simulink model "application"  (R2021b)
settings: Solver=FixedStepAuto  StartTime=0.0  StopTime=10.0  FixedStep=sampleTime  RelTol=1e-3
undefined symbols (not defined in the file or in its folder): AEMACE10_STBY, AEMACE8_STBY
libraries: simulink x10, EMACE_APP x6, AIL_STATE_MACHINE_LIB x2, AEMACE10_IN x1, AEMACE10_INSTRUMENTATION x1, AEMACE10_OUT x1, AEMACE8_IN x1, AEMACE8_INSTRUMENTATION x1, AEMACE8_OUT x1, SEMACE1_IN x1, SEMACE1_INSTRUMENTATION x1, SEMACE1_OUT x1
(part 2 of 2)

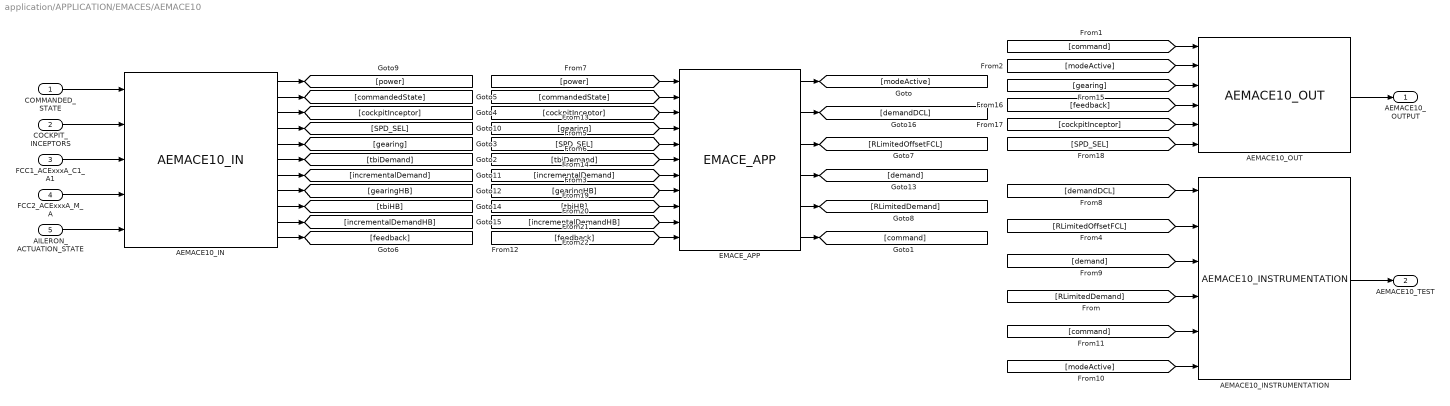
== system application/APPLICATION/EMACES/AEMACE10 ==
  COMMANDED_STATE : Inport
  COCKPIT_INCEPTORS : Inport  Port=2
  FCC1_ACExxxA_C1_A1 : Inport  Port=3
  FCC2_ACExxxA_M_A : Inport  Port=4
  AILERON_ACTUATION_STATE : Inport  Port=5
  AEMACE10_IN : AEMACE10_IN/AEMACE10_IN  SystemSampleTime=-1  VariantActivationTime=update diagram  Latency=0  AutoFrameSizeCalculation=off
  AEMACE10_INSTRUMENTATION : AEMACE10_INSTRUMENTATION/AEMACE10_INSTRUMENTATION  SystemSampleTime=-1  VariantActivationTime=update diagram  Latency=0  AutoFrameSizeCalculation=off
  AEMACE10_OUT : AEMACE10_OUT/AEMACE10_OUT  SystemSampleTime=-1  VariantActivationTime=update diagram  Latency=0  AutoFrameSizeCalculation=off
  EMACE_APP : EMACE_APP/EMACE_APP  SystemSampleTime=-1  VariantActivationTime=update diagram  Latency=0  AutoFrameSizeCalculation=off
      link override From10: GotoTag=command
  AEMACE10_OUTPUT : Outport
  AEMACE10_TEST : Outport  Port=2
  wires:
  COMMANDED_STATE/1 -> AEMACE10_IN/1
  COCKPIT_INCEPTORS/1 -> AEMACE10_IN/2
  FCC1_ACExxxA_C1_A1/1 -> AEMACE10_IN/3
  AILERON_ACTUATION_STATE/1 -> AEMACE10_IN/5
  [command] -> AEMACE10_OUT/1
  [modeActive] -> AEMACE10_OUT/2
  AEMACE10_OUT/1 -> AEMACE10_OUTPUT/1
  [demandDCL] -> AEMACE10_INSTRUMENTATION/1
  AEMACE10_INSTRUMENTATION/1 -> AEMACE10_TEST/1
  EMACE_APP/1 -> [modeActive]
  EMACE_APP/2 -> [demandDCL]
  EMACE_APP/6 -> [command]
  EMACE_APP/4 -> [demand]
  EMACE_APP/3 -> [RLimitedOffsetFCL]
  EMACE_APP/5 -> [RLimitedDemand]
  [modeActive] -> AEMACE10_INSTRUMENTATION/6
  [command] -> AEMACE10_INSTRUMENTATION/5
  [RLimitedDemand] -> AEMACE10_INSTRUMENTATION/4
  [demand] -> AEMACE10_INSTRUMENTATION/3
  [RLimitedOffsetFCL] -> AEMACE10_INSTRUMENTATION/2
  AEMACE10_IN/1 -> [power]
  AEMACE10_IN/4 -> [SPD_SEL]
  AEMACE10_IN/5 -> [gearing]
  AEMACE10_IN/6 -> [tbiDemand]
  AEMACE10_IN/11 -> [feedback]
  AEMACE10_IN/2 -> [commandedState]
  AEMACE10_IN/3 -> [cockpitInceptor]
  [power] -> EMACE_APP/1
  [commandedState] -> EMACE_APP/2
  [cockpitInceptor] -> EMACE_APP/3
  [gearing] -> EMACE_APP/4
  [SPD_SEL] -> EMACE_APP/5
  [tbiDemand] -> EMACE_APP/6
  [feedback] -> EMACE_APP/11
  [gearing] -> AEMACE10_OUT/3
  [feedback] -> AEMACE10_OUT/4
  [cockpitInceptor] -> AEMACE10_OUT/5
  [SPD_SEL] -> AEMACE10_OUT/6
  FCC2_ACExxxA_M_A/1 -> AEMACE10_IN/4
  AEMACE10_IN/7 -> [incrementalDemand]
  AEMACE10_IN/8 -> [gearingHB]
  AEMACE10_IN/9 -> [tbiHB]
  AEMACE10_IN/10 -> [incrementalDemandHB]
  [incrementalDemand] -> EMACE_APP/7
  [gearingHB] -> EMACE_APP/8
  [incrementalDemandHB] -> EMACE_APP/10
  [tbiHB] -> EMACE_APP/9

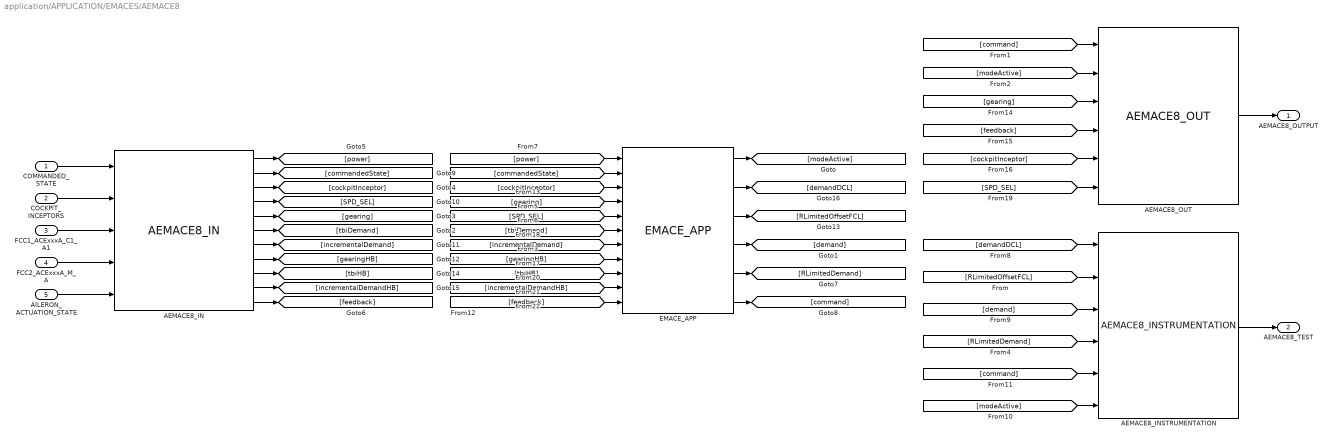
== system application/APPLICATION/EMACES/AEMACE8 ==
  COMMANDED_STATE : Inport
  COCKPIT_INCEPTORS : Inport  Port=2
  FCC1_ACExxxA_C1_A1 : Inport  Port=3
  FCC2_ACExxxA_M_A : Inport  Port=4
  AILERON_ACTUATION_STATE : Inport  Port=5
  AEMACE8_IN : AEMACE8_IN/AEMACE8_IN  SystemSampleTime=-1  VariantActivationTime=update diagram  Latency=0  AutoFrameSizeCalculation=off
      link override Rate Limiter: RisingSlewLimit=dataAEMACE.rateLimiterGearing  FallingSlewLimit=-dataAEMACE.rateLimiterGearing
  AEMACE8_INSTRUMENTATION : AEMACE8_INSTRUMENTATION/AEMACE8_INSTRUMENTATION  SystemSampleTime=-1  VariantActivationTime=update diagram  Latency=0  AutoFrameSizeCalculation=off
  AEMACE8_OUT : AEMACE8_OUT/AEMACE8_OUT  SystemSampleTime=-1  VariantActivationTime=update diagram  Latency=0  AutoFrameSizeCalculation=off
  EMACE_APP : EMACE_APP/EMACE_APP  SystemSampleTime=-1  VariantActivationTime=update diagram  Latency=0  AutoFrameSizeCalculation=off
  AEMACE8_OUTPUT : Outport
  AEMACE8_TEST : Outport  Port=2
  wires:
  COMMANDED_STATE/1 -> AEMACE8_IN/1
  COCKPIT_INCEPTORS/1 -> AEMACE8_IN/2
  FCC1_ACExxxA_C1_A1/1 -> AEMACE8_IN/3
  AILERON_ACTUATION_STATE/1 -> AEMACE8_IN/5
  AEMACE8_OUT/1 -> AEMACE8_OUTPUT/1
  [demandDCL] -> AEMACE8_INSTRUMENTATION/1
  AEMACE8_INSTRUMENTATION/1 -> AEMACE8_TEST/1
  EMACE_APP/1 -> [modeActive]
  EMACE_APP/2 -> [demandDCL]
  EMACE_APP/3 -> [RLimitedOffsetFCL]
  EMACE_APP/4 -> [demand]
  EMACE_APP/5 -> [RLimitedDemand]
  EMACE_APP/6 -> [command]
  [RLimitedOffsetFCL] -> AEMACE8_INSTRUMENTATION/2
  [demand] -> AEMACE8_INSTRUMENTATION/3
  [RLimitedDemand] -> AEMACE8_INSTRUMENTATION/4
  [command] -> AEMACE8_INSTRUMENTATION/5
  [modeActive] -> AEMACE8_INSTRUMENTATION/6
  [power] -> EMACE_APP/1
  [commandedState] -> EMACE_APP/2
  [cockpitInceptor] -> EMACE_APP/3
  [gearing] -> EMACE_APP/4
  [command] -> AEMACE8_OUT/1
  [modeActive] -> AEMACE8_OUT/2
  [gearing] -> AEMACE8_OUT/3
  [feedback] -> AEMACE8_OUT/4
  [cockpitInceptor] -> AEMACE8_OUT/5
  [SPD_SEL] -> EMACE_APP/5
  [tbiDemand] -> EMACE_APP/6
  [feedback] -> EMACE_APP/11
  [SPD_SEL] -> AEMACE8_OUT/6
  FCC2_ACExxxA_M_A/1 -> AEMACE8_IN/4
  AEMACE8_IN/1 -> [power]
  AEMACE8_IN/2 -> [commandedState]
  AEMACE8_IN/3 -> [cockpitInceptor]
  AEMACE8_IN/4 -> [SPD_SEL]
  AEMACE8_IN/5 -> [gearing]
  AEMACE8_IN/6 -> [tbiDemand]
  AEMACE8_IN/11 -> [feedback]
  AEMACE8_IN/7 -> [incrementalDemand]
  AEMACE8_IN/8 -> [gearingHB]
  AEMACE8_IN/9 -> [tbiHB]
  AEMACE8_IN/10 -> [incrementalDemandHB]
  [incrementalDemand] -> EMACE_APP/7
  [gearingHB] -> EMACE_APP/8
  [tbiHB] -> EMACE_APP/9
  [incrementalDemandHB] -> EMACE_APP/10

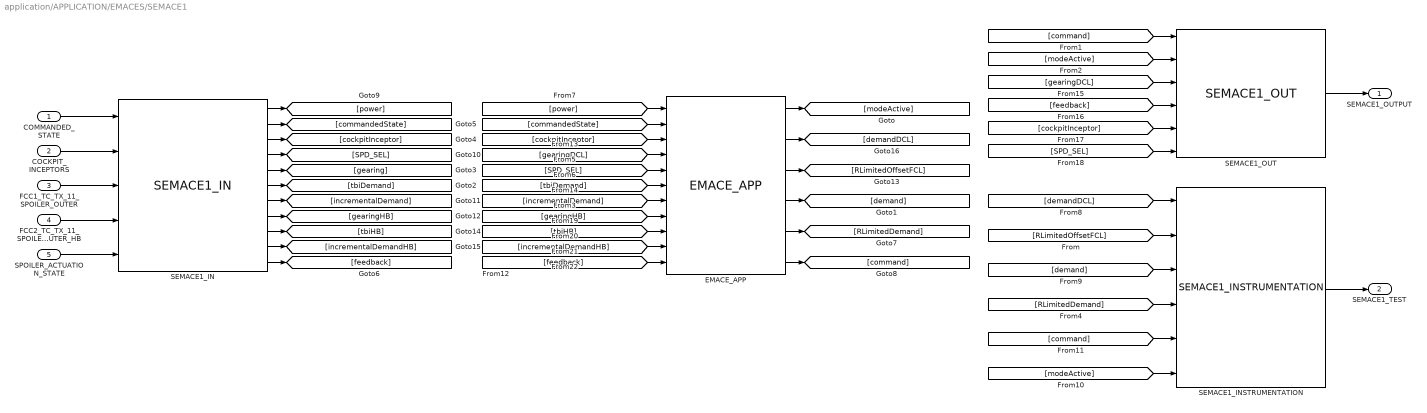
== system application/APPLICATION/EMACES/SEMACE1 ==
  COMMANDED_STATE : Inport
  COCKPIT_INCEPTORS : Inport  Port=2
  FCC1_TC_TX_11_SPOILER_OUTER : Inport  Port=3  OutDataTypeStr=Bus: FCC1_TC_TX_11_SPOILER_OUTER
  FCC2_TC_TX_11_SPOILER_OUTER_HB : Inport  Port=4  OutDataTypeStr=Bus: FCC2_TC_TX_11_SPOILER_OUTER_HB
  SPOILER_ACTUATION_STATE : Inport  Port=5  OutDataTypeStr=Bus: SPOILER_ACTUATION_STATE
  EMACE_APP : EMACE_APP/EMACE_APP  SystemSampleTime=-1  VariantActivationTime=update diagram  Latency=0  AutoFrameSizeCalculation=off
  SEMACE1_IN : SEMACE1_IN/SEMACE1_IN  SystemSampleTime=-1  VariantActivationTime=update diagram  Latency=0  AutoFrameSizeCalculation=off
  SEMACE1_INSTRUMENTATION : SEMACE1_INSTRUMENTATION/SEMACE1_INSTRUMENTATION  SystemSampleTime=-1  VariantActivationTime=update diagram  Latency=0  AutoFrameSizeCalculation=off
  SEMACE1_OUT : SEMACE1_OUT/SEMACE1_OUT  SystemSampleTime=-1  VariantActivationTime=update diagram  Latency=0  AutoFrameSizeCalculation=off
  SEMACE1_OUTPUT : Outport
  SEMACE1_TEST : Outport  Port=2
  wires:
  COMMANDED_STATE/1 -> SEMACE1_IN/1
  COCKPIT_INCEPTORS/1 -> SEMACE1_IN/2
  FCC1_TC_TX_11_SPOILER_OUTER/1 -> SEMACE1_IN/3
  SPOILER_ACTUATION_STATE/1 -> SEMACE1_IN/5
  [command] -> SEMACE1_OUT/1
  [modeActive] -> SEMACE1_OUT/2
  SEMACE1_OUT/1 -> SEMACE1_OUTPUT/1
  [demandDCL] -> SEMACE1_INSTRUMENTATION/1
  SEMACE1_INSTRUMENTATION/1 -> SEMACE1_TEST/1
  EMACE_APP/1 -> [modeActive]
  EMACE_APP/2 -> [demandDCL]
  EMACE_APP/3 -> [RLimitedOffsetFCL]
  EMACE_APP/4 -> [demand]
  EMACE_APP/5 -> [RLimitedDemand]
  EMACE_APP/6 -> [command]
  [RLimitedOffsetFCL] -> SEMACE1_INSTRUMENTATION/2
  [demand] -> SEMACE1_INSTRUMENTATION/3
  [RLimitedDemand] -> SEMACE1_INSTRUMENTATION/4
  [command] -> SEMACE1_INSTRUMENTATION/5
  [modeActive] -> SEMACE1_INSTRUMENTATION/6
  SEMACE1_IN/4 -> [SPD_SEL]
  SEMACE1_IN/5 -> [gearing]
  SEMACE1_IN/6 -> [tbiDemand]
  SEMACE1_IN/11 -> [feedback]
  SEMACE1_IN/1 -> [power]
  SEMACE1_IN/2 -> [commandedState]
  SEMACE1_IN/3 -> [cockpitInceptor]
  [power] -> EMACE_APP/1
  [commandedState] -> EMACE_APP/2
  [cockpitInceptor] -> EMACE_APP/3
  [gearingDCL] -> EMACE_APP/4
  [SPD_SEL] -> EMACE_APP/5
  [tbiDemand] -> EMACE_APP/6
  [feedback] -> EMACE_APP/11
  [gearingDCL] -> SEMACE1_OUT/3
  [feedback] -> SEMACE1_OUT/4
  [cockpitInceptor] -> SEMACE1_OUT/5
  [SPD_SEL] -> SEMACE1_OUT/6
  FCC2_TC_TX_11_SPOILER_OUTER_HB/1 -> SEMACE1_IN/4
  SEMACE1_IN/7 -> [incrementalDemand]
  SEMACE1_IN/8 -> [gearingHB]
  SEMACE1_IN/9 -> [tbiHB]
  SEMACE1_IN/10 -> [incrementalDemandHB]
  [incrementalDemandHB] -> EMACE_APP/10
  [tbiHB] -> EMACE_APP/9
  [gearingHB] -> EMACE_APP/8
  [incrementalDemand] -> EMACE_APP/7

== system application/APPLICATION/EMACES/SEMACE2 ==
  COMMANDED_STATE : Inport
  COCKPIT_INCEPTORS : Inport  Port=2
  FCC1_TC_TX_12_SPOILER_INNER : Inport  Port=3  OutDataTypeStr=Bus: FCC1_TC_TX_12_SPOILER_INNER
  FCC2_TC_TX_12_SPOILER_INNER_HB : Inport  Port=4  OutDataTypeStr=Bus: FCC2_TC_TX_12_SPOILER_INNER_HB
  SPOILER_ACTUATION_STATE : Inport  Port=5  OutDataTypeStr=Bus: SPOILER_ACTUATION_STATE
  EMACE_APP : EMACE_APP/EMACE_APP  SystemSampleTime=-1  VariantActivationTime=update diagram  Latency=0  AutoFrameSizeCalculation=off
  SEMACE2_IN : SEMACE2_IN/SEMACE2_IN  SystemSampleTime=-1  VariantActivationTime=update diagram  Latency=0  AutoFrameSizeCalculation=off
  SEMACE2_INSTRUMENTATION : SEMACE2_INSTRUMENTATION/SEMACE2_INSTRUMENTATION  SystemSampleTime=-1  VariantActivationTime=update diagram  Latency=0  AutoFrameSizeCalculation=off
  SEMACE2_OUT : SEMACE2_OUT/SEMACE2_OUT  SystemSampleTime=-1  VariantActivationTime=update diagram  Latency=0  AutoFrameSizeCalculation=off
  SEMACE2_OUTPUT : Outport
  SEMACE2_TEST : Outport  Port=2
  wires:
  [modeActive] -> SEMACE2_INSTRUMENTATION/6
  [command] -> SEMACE2_INSTRUMENTATION/5
  [RLimitedDemand] -> SEMACE2_INSTRUMENTATION/4
  [demand] -> SEMACE2_INSTRUMENTATION/3
  [RLimitedOffsetFCL] -> SEMACE2_INSTRUMENTATION/2
  EMACE_APP/6 -> [command]
  EMACE_APP/5 -> [RLimitedDemand]
  EMACE_APP/4 -> [demand]
  EMACE_APP/3 -> [RLimitedOffsetFCL]
  EMACE_APP/2 -> [demandDCL]
  EMACE_APP/1 -> [modeActive]
  SEMACE2_INSTRUMENTATION/1 -> SEMACE2_TEST/1
  [demandDCL] -> SEMACE2_INSTRUMENTATION/1
  SEMACE2_OUT/1 -> SEMACE2_OUTPUT/1
  [modeActive] -> SEMACE2_OUT/2
  [command] -> SEMACE2_OUT/1
  SPOILER_ACTUATION_STATE/1 -> SEMACE2_IN/5
  FCC1_TC_TX_12_SPOILER_INNER/1 -> SEMACE2_IN/3
  COCKPIT_INCEPTORS/1 -> SEMACE2_IN/2
  COMMANDED_STATE/1 -> SEMACE2_IN/1
  SEMACE2_IN/7 -> [feedback]
  SEMACE2_IN/1 -> [power]
  SEMACE2_IN/2 -> [commandedState]
  SEMACE2_IN/3 -> [cockpitInceptor]
  SEMACE2_IN/4 -> [SPD_SEL]
  SEMACE2_IN/5 -> [gearingDCL]
  SEMACE2_IN/6 -> [offsetFCL]
  [power] -> EMACE_APP/1
  [commandedState] -> EMACE_APP/2
  [cockpitInceptor] -> EMACE_APP/3
  [gearingDCL] -> EMACE_APP/4
  [SPD_SEL] -> EMACE_APP/5
  [offsetFCL] -> EMACE_APP/6
  [feedback] -> EMACE_APP/7
  [gearingDCL] -> SEMACE2_OUT/3
  [feedback] -> SEMACE2_OUT/4
  [cockpitInceptor] -> SEMACE2_OUT/5
  [SPD_SEL] -> SEMACE2_OUT/6
  FCC2_TC_TX_12_SPOILER_INNER_HB/1 -> SEMACE2_IN/4

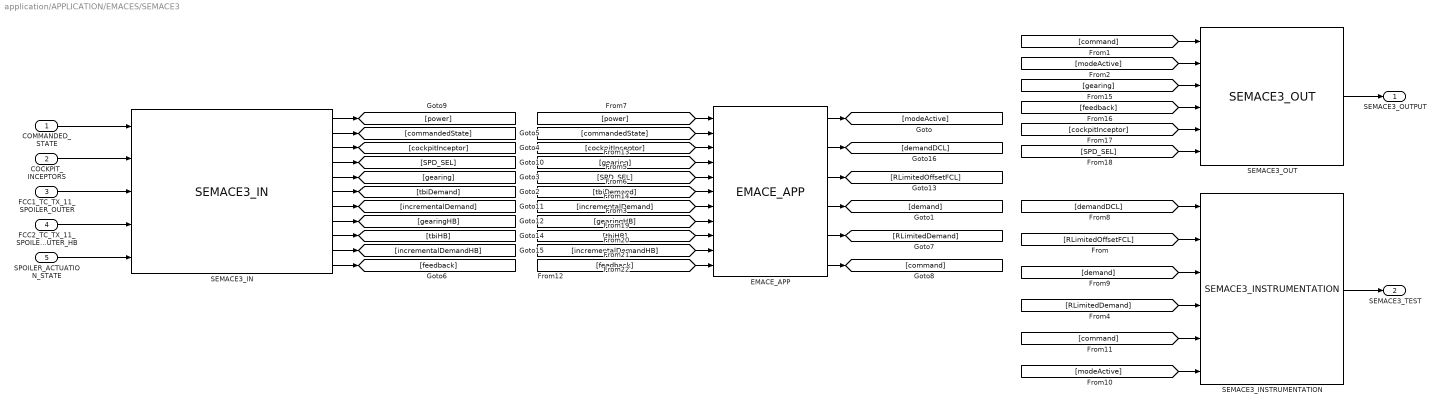
== system application/APPLICATION/EMACES/SEMACE3 ==
  COMMANDED_STATE : Inport
  COCKPIT_INCEPTORS : Inport  Port=2
  FCC1_TC_TX_11_SPOILER_OUTER : Inport  Port=3  OutDataTypeStr=Bus: FCC1_TC_TX_11_SPOILER_OUTER
  FCC2_TC_TX_11_SPOILER_OUTER_HB : Inport  Port=4  OutDataTypeStr=Bus: FCC2_TC_TX_11_SPOILER_OUTER_HB
  SPOILER_ACTUATION_STATE : Inport  Port=5  OutDataTypeStr=Bus: SPOILER_ACTUATION_STATE
  EMACE_APP : EMACE_APP/EMACE_APP  SystemSampleTime=-1  VariantActivationTime=update diagram  Latency=0  AutoFrameSizeCalculation=off
  SEMACE3_IN : SEMACE3_IN/SEMACE3_IN  SystemSampleTime=-1  VariantActivationTime=update diagram  Latency=0  AutoFrameSizeCalculation=off
  SEMACE3_INSTRUMENTATION : SEMACE3_INSTRUMENTATION/SEMACE3_INSTRUMENTATION  SystemSampleTime=-1  VariantActivationTime=update diagram  Latency=0  AutoFrameSizeCalculation=off
  SEMACE3_OUT : SEMACE3_OUT/SEMACE3_OUT  SystemSampleTime=-1  VariantActivationTime=update diagram  Latency=0  AutoFrameSizeCalculation=off
  SEMACE3_OUTPUT : Outport
  SEMACE3_TEST : Outport  Port=2
  wires:
  [modeActive] -> SEMACE3_INSTRUMENTATION/6
  [command] -> SEMACE3_INSTRUMENTATION/5
  [RLimitedDemand] -> SEMACE3_INSTRUMENTATION/4
  [demand] -> SEMACE3_INSTRUMENTATION/3
  [RLimitedOffsetFCL] -> SEMACE3_INSTRUMENTATION/2
  EMACE_APP/6 -> [command]
  EMACE_APP/5 -> [RLimitedDemand]
  EMACE_APP/4 -> [demand]
  EMACE_APP/3 -> [RLimitedOffsetFCL]
  EMACE_APP/2 -> [demandDCL]
  EMACE_APP/1 -> [modeActive]
  SEMACE3_INSTRUMENTATION/1 -> SEMACE3_TEST/1
  [demandDCL] -> SEMACE3_INSTRUMENTATION/1
  SEMACE3_OUT/1 -> SEMACE3_OUTPUT/1
  [modeActive] -> SEMACE3_OUT/2
  [command] -> SEMACE3_OUT/1
  SPOILER_ACTUATION_STATE/1 -> SEMACE3_IN/5
  FCC1_TC_TX_11_SPOILER_OUTER/1 -> SEMACE3_IN/3
  COCKPIT_INCEPTORS/1 -> SEMACE3_IN/2
  COMMANDED_STATE/1 -> SEMACE3_IN/1
  SEMACE3_IN/11 -> [feedback]
  SEMACE3_IN/1 -> [power]
  SEMACE3_IN/2 -> [commandedState]
  SEMACE3_IN/3 -> [cockpitInceptor]
  SEMACE3_IN/4 -> [SPD_SEL]
  SEMACE3_IN/5 -> [gearing]
  SEMACE3_IN/6 -> [tbiDemand]
  [power] -> EMACE_APP/1
  [commandedState] -> EMACE_APP/2
  [cockpitInceptor] -> EMACE_APP/3
  [gearing] -> EMACE_APP/4
  [SPD_SEL] -> EMACE_APP/5
  [tbiDemand] -> EMACE_APP/6
  [feedback] -> EMACE_APP/11
  [gearing] -> SEMACE3_OUT/3
  [feedback] -> SEMACE3_OUT/4
  [cockpitInceptor] -> SEMACE3_OUT/5
  [SPD_SEL] -> SEMACE3_OUT/6
  FCC2_TC_TX_11_SPOILER_OUTER_HB/1 -> SEMACE3_IN/4
  SEMACE3_IN/7 -> [incrementalDemand]
  SEMACE3_IN/8 -> [gearingHB]
  SEMACE3_IN/9 -> [tbiHB]
  SEMACE3_IN/10 -> [incrementalDemandHB]
  [incrementalDemand] -> EMACE_APP/7
  [gearingHB] -> EMACE_APP/8
  [tbiHB] -> EMACE_APP/9
  [incrementalDemandHB] -> EMACE_APP/10

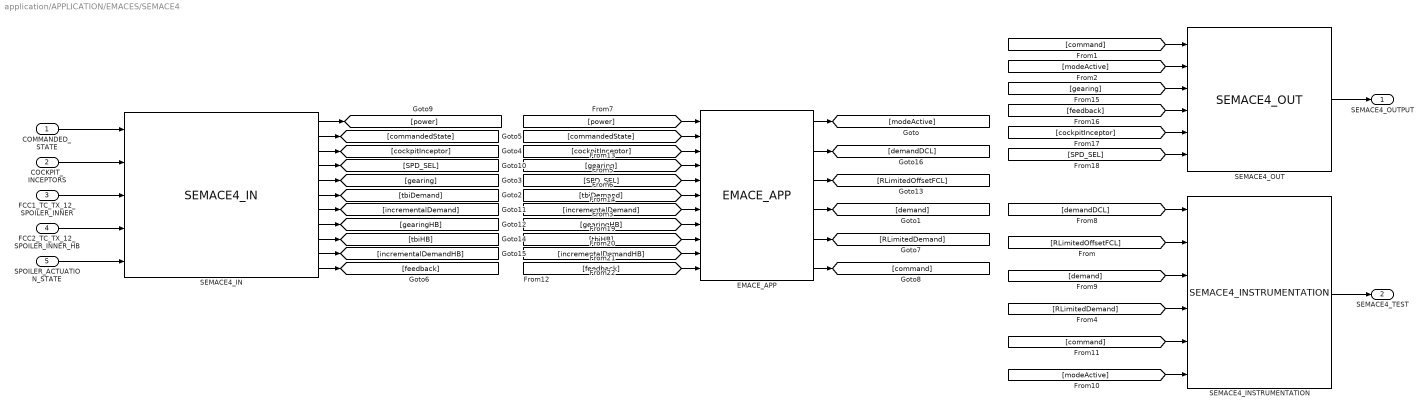
== system application/APPLICATION/EMACES/SEMACE4 ==
  COMMANDED_STATE : Inport
  COCKPIT_INCEPTORS : Inport  Port=2
  FCC1_TC_TX_12_SPOILER_INNER : Inport  Port=3  OutDataTypeStr=Bus: FCC1_TC_TX_12_SPOILER_INNER
  FCC2_TC_TX_12_SPOILER_INNER_HB : Inport  Port=4  OutDataTypeStr=Bus: FCC2_TC_TX_12_SPOILER_INNER_HB
  SPOILER_ACTUATION_STATE : Inport  Port=5  OutDataTypeStr=Bus: SPOILER_ACTUATION_STATE
  EMACE_APP : EMACE_APP/EMACE_APP  SystemSampleTime=-1  VariantActivationTime=update diagram  Latency=0  AutoFrameSizeCalculation=off
  SEMACE4_IN : SEMACE4_IN/SEMACE4_IN  SystemSampleTime=-1  VariantActivationTime=update diagram  Latency=0  AutoFrameSizeCalculation=off
  SEMACE4_INSTRUMENTATION : SEMACE4_INSTRUMENTATION/SEMACE4_INSTRUMENTATION  SystemSampleTime=-1  VariantActivationTime=update diagram  Latency=0  AutoFrameSizeCalculation=off
  SEMACE4_OUT : SEMACE4_OUT/SEMACE4_OUT  SystemSampleTime=-1  VariantActivationTime=update diagram  Latency=0  AutoFrameSizeCalculation=off
  SEMACE4_OUTPUT : Outport
  SEMACE4_TEST : Outport  Port=2
  wires:
  COMMANDED_STATE/1 -> SEMACE4_IN/1
  COCKPIT_INCEPTORS/1 -> SEMACE4_IN/2
  FCC1_TC_TX_12_SPOILER_INNER/1 -> SEMACE4_IN/3
  SPOILER_ACTUATION_STATE/1 -> SEMACE4_IN/5
  [command] -> SEMACE4_OUT/1
  [modeActive] -> SEMACE4_OUT/2
  SEMACE4_OUT/1 -> SEMACE4_OUTPUT/1
  [demandDCL] -> SEMACE4_INSTRUMENTATION/1
  SEMACE4_INSTRUMENTATION/1 -> SEMACE4_TEST/1
  EMACE_APP/1 -> [modeActive]
  EMACE_APP/2 -> [demandDCL]
  EMACE_APP/3 -> [RLimitedOffsetFCL]
  EMACE_APP/4 -> [demand]
  EMACE_APP/5 -> [RLimitedDemand]
  EMACE_APP/6 -> [command]
  [RLimitedOffsetFCL] -> SEMACE4_INSTRUMENTATION/2
  [demand] -> SEMACE4_INSTRUMENTATION/3
  [RLimitedDemand] -> SEMACE4_INSTRUMENTATION/4
  [command] -> SEMACE4_INSTRUMENTATION/5
  [modeActive] -> SEMACE4_INSTRUMENTATION/6
  SEMACE4_IN/3 -> [cockpitInceptor]
  SEMACE4_IN/4 -> [SPD_SEL]
  SEMACE4_IN/5 -> [gearing]
  SEMACE4_IN/6 -> [tbiDemand]
  SEMACE4_IN/11 -> [feedback]
  SEMACE4_IN/1 -> [power]
  SEMACE4_IN/2 -> [commandedState]
  [power] -> EMACE_APP/1
  [commandedState] -> EMACE_APP/2
  [cockpitInceptor] -> EMACE_APP/3
  [gearing] -> EMACE_APP/4
  [SPD_SEL] -> EMACE_APP/5
  [tbiDemand] -> EMACE_APP/6
  [feedback] -> EMACE_APP/11
  [gearing] -> SEMACE4_OUT/3
  [feedback] -> SEMACE4_OUT/4
  [cockpitInceptor] -> SEMACE4_OUT/5
  [SPD_SEL] -> SEMACE4_OUT/6
  FCC2_TC_TX_12_SPOILER_INNER_HB/1 -> SEMACE4_IN/4
  SEMACE4_IN/7 -> [incrementalDemand]
  SEMACE4_IN/8 -> [gearingHB]
  SEMACE4_IN/9 -> [tbiHB]
  SEMACE4_IN/10 -> [incrementalDemandHB]
  [incrementalDemand] -> EMACE_APP/7
  [gearingHB] -> EMACE_APP/8
  [tbiHB] -> EMACE_APP/9
  [incrementalDemandHB] -> EMACE_APP/10

== system application/APPLICATION/Subsystem/GENERATOR_STATE_CMD_LH_AIL ==
  LH_AIL_STATE : Inport
  Compare To Constant : simulink/Logic and Bit Operations/Compare To Constant  relop===  const=2  OutDataTypeStr=boolean
  Compare To Constant3 : simulink/Logic and Bit Operations/Compare To Constant  relop===  const=1  OutDataTypeStr=boolean
  Compare To Constant6 : simulink/Logic and Bit Operations/Compare To Constant  relop===  const=1  OutDataTypeStr=boolean
  Compare To Constant7 : simulink/Logic and Bit Operations/Compare To Constant  relop===  const=2  OutDataTypeStr=boolean
  Constant : Constant  OutDataTypeStr=boolean
  Constant1 : Constant  Value=0  OutDataTypeStr=boolean
  Constant2 : Constant  OutDataTypeStr=boolean
  Constant3 : Constant  Value=0  OutDataTypeStr=boolean
  Delay2 : Delay  DelayLength=1
  Delay3 : Delay  DelayLength=1
  Switch{,1..3} (4 alike) : Switch  Criteria=u2 > Threshold
  AEMACE8_CMD_STATE : Outport
  ACE9_CMD_STATE : Outport  Port=2
  wires:
  Constant/1 -> Switch/1
  Compare To Constant6/1 -> Switch2/2
  Switch/1 -> AEMACE8_CMD_STATE/1, Delay2/1
  Compare To Constant/1 -> Switch/2
  LH_AIL_STATE/1 -> Compare To Constant7/1, Compare To Constant6/1, Compare To Constant3/1, Compare To Constant/1
  Delay2/1 -> Switch1/3
  Switch1/1 -> Switch/3
  Constant3/1 -> Switch3/1
  Switch2/1 -> ACE9_CMD_STATE/1, Delay3/1
  Delay3/1 -> Switch3/3
  Constant2/1 -> Switch2/1
  Compare To Constant7/1 -> Switch3/2
  Switch3/1 -> Switch2/3
  Compare To Constant3/1 -> Switch1/2
  Constant1/1 -> Switch1/1

== system application/APPLICATION/Subsystem/GENERATOR_STATE_CMD_RH_AIL ==
  LH_AIL_STATE : Inport
  Compare To Constant : simulink/Logic and Bit Operations/Compare To Constant  relop===  const=2  OutDataTypeStr=boolean
  Compare To Constant3 : simulink/Logic and Bit Operations/Compare To Constant  relop===  const=1  OutDataTypeStr=boolean
  Compare To Constant6 : simulink/Logic and Bit Operations/Compare To Constant  relop===  const=1  OutDataTypeStr=boolean
  Compare To Constant7 : simulink/Logic and Bit Operations/Compare To Constant  relop===  const=2  OutDataTypeStr=boolean
  Constant : Constant  OutDataTypeStr=boolean
  Constant1 : Constant  Value=0  OutDataTypeStr=boolean
  Constant2 : Constant  OutDataTypeStr=boolean
  Constant3 : Constant  Value=0  OutDataTypeStr=boolean
  Delay2 : Delay  DelayLength=1
  Delay3 : Delay  DelayLength=1
  Switch{,1..3} (4 alike) : Switch  Criteria=u2 > Threshold
  AEMACE10_CMD_STATE : Outport
  ACE11_CMD_STATE : Outport  Port=2
  wires:
  Constant1/1 -> Switch1/1
  Compare To Constant3/1 -> Switch1/2
  Switch3/1 -> Switch2/3
  Compare To Constant7/1 -> Switch3/2
  Constant2/1 -> Switch2/1
  Delay3/1 -> Switch3/3
  Switch2/1 -> Delay3/1, ACE11_CMD_STATE/1
  Constant3/1 -> Switch3/1
  Switch1/1 -> Switch/3
  Delay2/1 -> Switch1/3
  LH_AIL_STATE/1 -> Compare To Constant/1, Compare To Constant3/1, Compare To Constant6/1, Compare To Constant7/1
  Compare To Constant/1 -> Switch/2
  Switch/1 -> Delay2/1, AEMACE10_CMD_STATE/1
  Compare To Constant6/1 -> Switch2/2
  Constant/1 -> Switch/1
